simulink model "wash2_test_question"  (R2024b)
settings: Solver=VariableStepAuto  StartTime=0.0  StopTime=inf  RelTol=1e-3
settings Model: Creator=kanith kumar  LastModifiedBy=kanith kumar

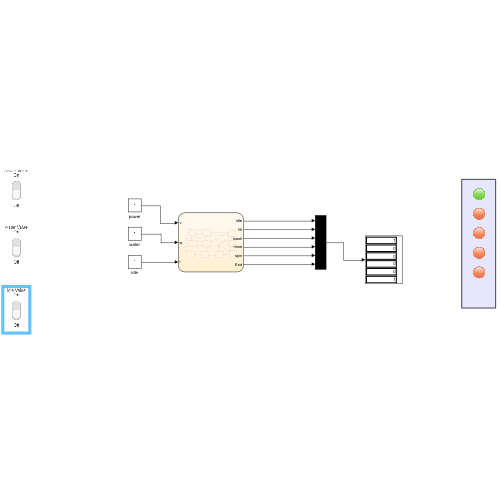
[thumbnail: Simulink's stored preview of the top-level diagram]
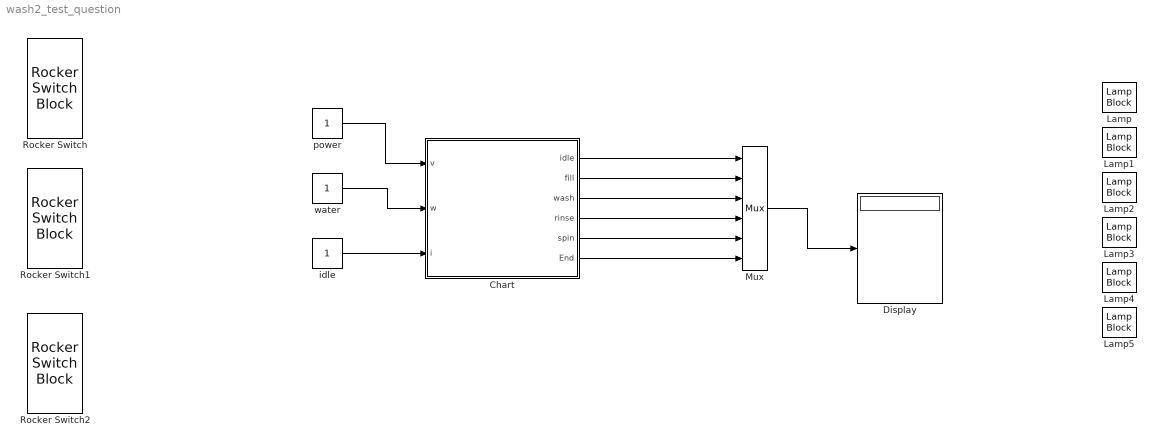
== system wash2_test_question ==
  Chart : Stateflow chart  TreatAsAtomicUnit=on
  Display : Display
  Lamp{,1..5} (6 alike) : LampBlock  LabelPosition=Hide
  Mux : Mux  Inputs=6
  Rocker Switch : RockerSwitchBlock
      settings: Values={{'Off', 'On'}, [0 1]}
  Rocker Switch1 : RockerSwitchBlock
      settings: Values={{'Off', 'On'}, [0 1]}
  Rocker Switch2 : RockerSwitchBlock
      settings: Values={{'Off', 'On'}, [0 1]}
  idle : Constant
  power : Constant
  water : Constant
  wires:
  Chart/1(idle) -> Mux/1
  Chart/2(fill) -> Mux/2
  Chart/3(wash) -> Mux/3
  Chart/4(rinse) -> Mux/4
  Chart/5(spin) -> Mux/5
  Chart/6(End) -> Mux/6
  Mux/1 -> Display/1
  power/1 -> Chart/1(v)
  water/1 -> Chart/2(w)
  idle/1 -> Chart/3(i)

== stateflow chart wash2_test_question/Chart ==
  state Power_off
    entry:
  state power_on
    entry:
  state idle
    entry:
    idle=1;
  state fill
    entry:
    during:
    fill=1
  state water_on
    entry:
  state water_off
    entry:
  state wash
    entry:
    fill=0;
    during:
    wash=1
  state End
    entry:
    spin=0;
    during:
    End=1;
  state spin
    entry:
    rinse=0;
    during:
    spin=1;
  state rinse
    entry:
    wash=0;
    during:
    rinse=1;
  (default) -> Power_off
  Power_off -> power_on : [v==1]
  idle -> power_on [order 1] : [i==1]
  water_on -> idle [order 3] : [i==1]
  power_on -> Power_off [order 1] : [v==0]
  (junction 50) -> idle
  water_off -> Power_off [order 2]
  power_on -> water_on [order 2]
  (junction 41) -> idle
  idle -> fill [order 2] : [i==0]
  fill -> idle [order 2] : [i==1]
  End -> (junction 50) : [i==1]
  water_off -> water_on [order 1] : [w==1]
  water_on -> fill [order 1] : [after(5,sec)]
  water_on -> water_off [order 2] : [w==0]
  spin -> (junction 41) [order 2] : [i==1]
  wash -> (junction 41) [order 2] : [i==1]
  rinse -> (junction 41) [order 2] : [i==1]
  fill -> wash [order 1] : [after(5,sec)]
  wash -> rinse [order 1] : [after(3,sec)]
  spin -> End [order 1] : [after(3,sec)]
  rinse -> spin [order 1] : [after(3,sec)]
  data: v input; w input; idle output; fill output; wash output; rinse output; spin output; End output; i input
